simulink model "GMSK_IQ_block"  (R2024a)
settings: Solver=FixedStepAuto  StartTime=0.0  StopTime=3e-5  FixedStep=1/9e9  RelTol=1e-3
values from neighbouring files (symbols this model uses):
  GTF_tap_coefficients = P(k)    [GTF_coef.m]
undefined symbols (not defined in the file or in its folder): DESIGN_CONST, DiscIntNeverNeededParam
settings Model: Creator=Sayantan  LastModifiedBy=Sayantan

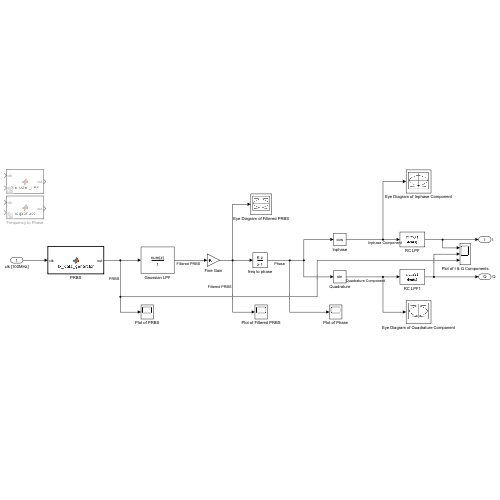
[thumbnail: Simulink's stored preview of the top-level diagram]
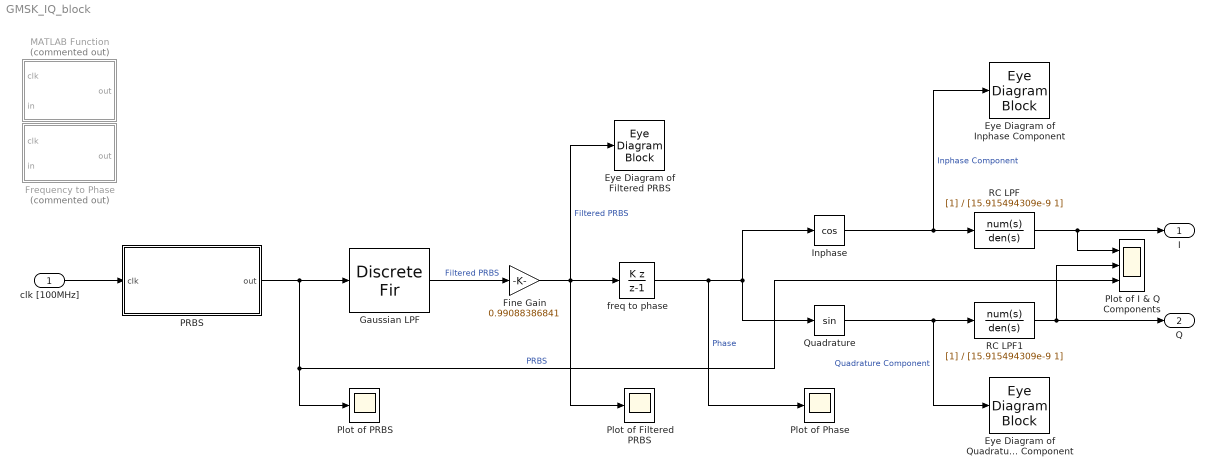
== system GMSK_IQ_block ==
  clk [100MHz] : Inport  SampleTime=DESIGN_CONST.Tsim
  Eye Diagram of Filtered PRBS : EyeDiagramBlock  WindowPosition=[2.000000,-36.000000,1366.000000,745.000000,]  ScopeFrameLocation=window  SamplesPerSymbol=100  TracesToDisplay=30  YLimits=[-7961857.402387202,7961857.402387202]  PlotImaginaryAxes=off
  Eye Diagram of Inphase Component : EyeDiagramBlock  WindowPosition=[-29.000000,-47.000000,1366.000000,745.000000,]  ScopeFrameLocation=window  SamplesPerSymbol=100  TracesToDisplay=15  YLimits=[-1.2499974903046622,1.249996338403037]  PlotImaginaryAxes=off
  Eye Diagram of Quadrature Component : EyeDiagramBlock  WindowPosition=[411.000000,16.000000,544.000000,736.000000,]  ScopeFrameLocation=window  SamplesPerSymbol=100  TracesToDisplay=15  YLimits=[-1.2499974903046622,1.249996338403037]  PlotImaginaryAxes=off
  Fine Gain : Gain  Gain=0.99088386841
  Frequency to Phase : MATLAB Function  Commented=on  TreatAsAtomicUnit=on  SystemSampleTime=DESIGN_CONST.Tsim
  Gaussian LPF : DiscreteFir  Coefficients=GTF_tap_coefficients
  Inphase : Trigonometry  Operator=cos
  MATLAB Function : MATLAB Function  Commented=on  TreatAsAtomicUnit=on  SystemSampleTime=DESIGN_CONST.Tsim
  PRBS : MATLAB Function  TreatAsAtomicUnit=on  SystemSampleTime=DESIGN_CONST.Tsim
  Plot of Filtered PRBS : Scope
  Plot of I & Q Components : Scope  NumInputPorts=3
  Plot of PRBS : Scope
  Plot of Phase : Scope
  Quadrature : Trigonometry
  RC LPF : TransferFcn  Denominator=[15.915494309e-9 1]
  RC LPF1 : TransferFcn  Denominator=[15.915494309e-9 1]
  freq to phase : DiscreteIntegrator  IntegratorMethod=Accumulation: Backward Euler  gainval=2 * pi * DESIGN_CONST.T  SampleTime=DESIGN_CONST.T  ICPrevOutput=DiscIntNeverNeededParam  ICPrevScaledInput=DiscIntNeverNeededParam
  I : Outport  SignalName=I
  Q : Outport  Port=2  SignalName=Q
  wires:
  clk [100MHz]/1 -> PRBS/1(clk)
  PRBS/1(out) -> Plot of PRBS/1, Plot of I & Q Components/3, Gaussian LPF/1  "PRBS"
  Gaussian LPF/1 -> Fine Gain/1  "Filtered PRBS"
  freq to phase/1 -> Quadrature/1, Inphase/1, Plot of Phase/1  "Phase"
  Inphase/1 -> Eye Diagram of Inphase Component/1, RC LPF/1  "Inphase Component"
  Fine Gain/1 -> Plot of Filtered PRBS/1, Eye Diagram of Filtered PRBS/1, freq to phase/1  "Filtered PRBS"
  Quadrature/1 -> Eye Diagram of Quadrature Component/1, RC LPF1/1  "Quadrature Component"
  RC LPF/1 -> Plot of I & Q Components/1, I/1
  RC LPF1/1 -> Q/1, Plot of I & Q Components/2

== matlab function GMSK_IQ_block/PRBS ==
  data: clk input; out output
function out = Tx_data_generator(clk)
%TX_DATA_GENERATOR Generates PRBS at data rate (1/Td) using Bernoulli

persistent output_value output_index clk_val

if isempty(clk_val)
    clk_val = 0;
end

if isempty(output_index) || (clk - clk_val == 1)
    if isempty(output_index)
        output_index = 0;
        output_value = repmat(randi([0 1])*2 - 1, [1 DESIGN_CONST.Td / DESIGN_CONST.T]);
    end
    if output_index == DESIGN_CONST.Td / DESIGN_CONST.T
        output_index = 0;
        output_value = repmat(randi([0 1])*2 - 1, [1 DESIGN_CONST.Td / DESIGN_CONST.T]);
    end
    output_index = output_index + 1;
end
clk_val = clk;

out = output_value(output_index);

end

== matlab function GMSK_IQ_block/Frequency to Phase ==
  data: clk input; out output; in input
function out = freq2phase(clk, in)

    Kph = 2*pi*DESIGN_CONST.T;
    
    persistent phase edge_detector

    if isempty(phase)
        phase = 0;
        edge_detector = CLK(clk);
    end

    if edge_detector.posedge(clk)
        phase = phase + in * Kph;
    end

    out = phase;
end

== matlab function GMSK_IQ_block/MATLAB Function ==
  data: clk input; out output; in input
function out = Gaussian_LPF(clk, in)
    
    persistent signal edge_detector k GTF_tap_coefficients

    if isempty(signal)
        % 5 sample periods
        k = 0 : DESIGN_CONST.T : 5 * DESIGN_CONST.Td;
        GTF_tap_coefficients = (DESIGN_CONST.T * DESIGN_CONST.h * exp(-k.^2/(2*DESIGN_CONST.SIGMA^2)) / (DESIGN_CONST.Td * DESIGN_CONST.SIGMA * sqrt(2*pi)));
        
        signal = zeros(size(k));
        edge_detector = CLK(clk);
    end

    if edge_detector.posedge(clk)
        signal = [in, signal(1:end-1)];
    end

    out = sum(signal .* GTF_tap_coefficients);
end
